simulink model "HSX_multi_fin"  (R2023b)
settings: Solver=VariableStepAuto  StartTime=0.0  StopTime=T_end  RelTol=1e-3
undefined symbols (not defined in the file): Kanti, Ki, Kp, LHSX, Ra, RHSX, T_trigger, Tdead, Ts, Tsamp, Vf
libraries: spsCurrentMeasurementLib x6, spsVoltageMeasurementLib x6, spsSeriesRLCBranchLib x6, spsMosfetLib x4, spsControlledVoltageSourceLib x2, spsDCMachineLib x2, spsSawtoothGeneratorLib x2, spsGroundLib x2, spsIdealSwitchLib x2, spsDCVoltageSourceLib x2, spsDiodeLib x1, sps_lib x1
settings Model: Creator=baik3-ad  LastModifiedBy=baik3-ad

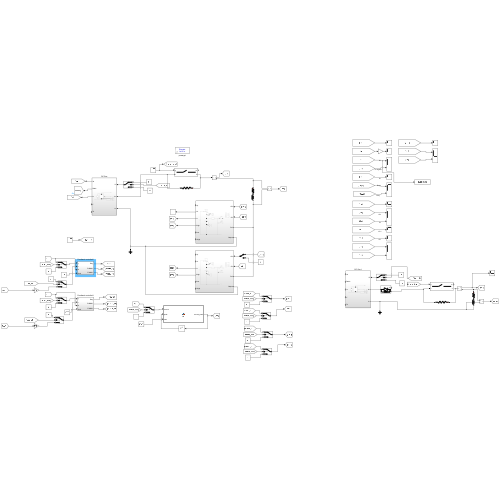
[thumbnail: Simulink's stored preview of the top-level diagram]
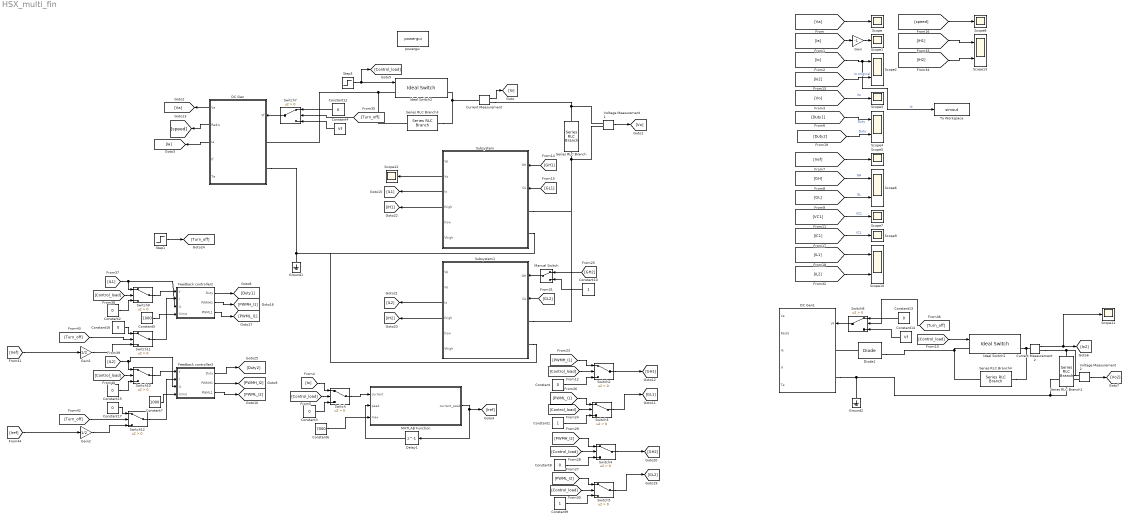
== system HSX_multi_fin ==
  Constant{,2..3,8,12..13,15..17} (9 alike) : Constant  Value=0
  Constant1 : Constant
  Constant10 : Constant
  Constant14 : Constant  Value=Vf
  Constant4 : Constant  Value=Vf
  Constant5 : Constant  Value=1000
  Constant6 : Constant  Value=7000
  Constant7 : Constant  Value=1000
  Constant9 : Constant
  Current Measurement : spsCurrentMeasurementLib/Current Measurement  PhasorSimulation=off  OutputType=Complex  PSBequivalent=0
  Current Measurement2 : spsCurrentMeasurementLib/Current Measurement  PhasorSimulation=off  OutputType=Complex  PSBequivalent=0
  DC Gen : Subsystem
  DC Gen1 : Subsystem
  Delay1 : Delay  DelayLength=1  InitialCondition=0  SampleTime=Tsamp
  Diode1 : spsDiodeLib/Diode  Ron=0.001  Lon=0  Vf=0.8  IC=0  UseSnubber=0  Rs=500  Cs=250e-9  Measurements=on
  Feedback controller2 : Subsystem
  Feedback controller3 : Subsystem
  Gain : Gain  Gain=-1
  Gain1 : Gain  Gain=1/2
  Gain2 : Gain  Gain=1/2
  Ground1 : spsGroundLib/Ground  LConnTagsString=a
  Ground2 : spsGroundLib/Ground  LConnTagsString=a
  Ideal Switch1 : spsIdealSwitchLib/Ideal Switch  Ron=1e-6  Lon=0  IC=0  Rs=1e8  Cs=0  Measurements=on
  Ideal Switch2 : spsIdealSwitchLib/Ideal Switch  Ron=1e-6  Lon=0  IC=0  Rs=1e8  Cs=0  Measurements=on
  MATLAB Function : MATLAB Function  TreatAsAtomicUnit=on
  Manual Switch : ManualSwitch
  Scope{,1,3,5,7..9,11..12} (9 alike) : Scope
  Scope{2,4,6,10,13} (5 alike) : Scope  NumInputPorts=2
  Series RLC Branch : spsSeriesRLCBranchLib/Series RLC Branch  LConnTagsString=__new0  RConnTagsString=__new0  BranchType=RL  Resistance=RHSX*10  Inductance=LHSX*10  SetiL0=off  InitialCurrent=0  Capacitance=1e-6  Setx0=off  InitialVoltage=0  Measurements=None
  Series RLC Branch1 : spsSeriesRLCBranchLib/Series RLC Branch  LConnTagsString=__new0  RConnTagsString=__new0  BranchType=RL  Resistance=RHSX*10  Inductance=LHSX*10  SetiL0=off  InitialCurrent=0  Capacitance=1e-6  Setx0=off  InitialVoltage=0  Measurements=None
  Series RLC Branch3 : spsSeriesRLCBranchLib/Series RLC Branch  LConnTagsString=__new0  RConnTagsString=__new0  BranchType=R  Resistance=1e8  Inductance=0  SetiL0=off  InitialCurrent=0  Capacitance=1e-6  Setx0=off  InitialVoltage=0  Measurements=None
  Series RLC Branch4 : spsSeriesRLCBranchLib/Series RLC Branch  LConnTagsString=__new0  RConnTagsString=__new0  BranchType=R  Resistance=1e8  Inductance=0  SetiL0=off  InitialCurrent=0  Capacitance=1e-6  Setx0=off  InitialVoltage=0  Measurements=None
  Step1 : Step  Time=T_trigger+1.5  SampleTime=0  VectorParams1D=off  ZeroCross=off
  Step3 : Step  Time=T_trigger  SampleTime=0  VectorParams1D=off  ZeroCross=off
  Subsystem : Subsystem
  Subsystem1 : Subsystem
  Switch{,2..5,7..12} (11 alike) : Switch  Criteria=u2 > Threshold  SaturateOnIntegerOverflow=off  InputSameDT=off
  To Workspace : ToWorkspace  VariableName=simout  SaveFormat=Timeseries  SampleTime=-1
  Voltage Measurement1 : spsVoltageMeasurementLib/Voltage Measurement  PhasorSimulation=off  OutputType=Complex  PSBequivalent=0
  Voltage Measurement2 : spsVoltageMeasurementLib/Voltage Measurement  PhasorSimulation=off  OutputType=Complex  PSBequivalent=0
  powergui : sps_lib/powergui  Priority=1  SimulationMode=Discrete  SampleTime=Tsamp  frequency=60  Iterations=50  frequencyindice=0  Pbase=100e6  ErrMax=1e-4  UnitsV=kV  UnitsW=MW  buscounter=0  FunctionMessages=off  echomessages=off  EnableUseOfTLC=off  CurrentSourceSwitches=off  DisableSnubberDevices=off  DisableRonSwitches=off  DisableVfSwitches=off  DisplayEquations=off  AutomaticDiscreteSolvers=off  SolverType=Tustin/Backward Euler (TBE)  Interpol=off  ExternalGateDelay=off  methode=off  Ts=100  x0status=blocks  SPID=on  SwTol=0  HookPort=off  NonlinearTolerance=1e-4  nMaxIteration=100  ContinueOnMaxIteration=off  RestoreLinks=warning  ResistiveCurrentMeasurement=off  Frange=[0:2:500]  Ylog=off  Xlog=on  ShowGrid=off  save=off  variable=ZData  structure=0  ZoomFFT=off  StartTime=0.0  cycles=1  DisplayStyle=1  fundamental=60  FreqAxis=off  MaxFrequency=1000  frequencyindicesteady=1  RmsSteady=1  display=off
  wires:
  Step3/1 -> [Control_load], Ideal Switch2/1
  Current Measurement/1 -> [Io]
  Voltage Measurement1/1 -> [Vo]
  [Va] -> Scope/1
  [Io] -> To Workspace/1, Scope2/1  "Io"
  [Vo] -> Scope3/1  "Vo"
  [Ia] -> Gain/1
  Gain/1 -> Scope1/1
  MATLAB Function/1(current_peak) -> [Iref], Delay1/1
  Delay1/1 -> MATLAB Function/2(peak)
  [Iref] -> Scope5/1
  [GH] -> Scope6/1  "GH"
  [GL] -> Scope6/2  "GL"
  [VC1] -> Scope7/1  "VC1"
  Switch2/1 -> [GH1]
  Switch3/1 -> [GL1]
  [speed] -> Scope8/1
  [IC1] -> Scope9/1  "IC1"
  [IL1] -> Scope10/1
  [Control_load] -> Switch/2
  Switch/1 -> MATLAB Function/1(current)
  [Io] -> Switch/1
  Constant3/1 -> Switch/3
  [Control_load] -> Switch2/2
  [PWMH_I1] -> Switch2/1
  Constant/1 -> Switch2/3
  [PWML_I1] -> Switch3/1
  Constant1/1 -> Switch3/3
  [Control_load] -> Switch3/2
  Current Measurement2/1 -> Scope11/1, [Io2]
  Voltage Measurement2/1 -> [Vo2]
  [Control_load] -> Ideal Switch1/1
  [Io2] -> Scope2/2  "Io original"
  [Duty1] -> Scope4/1  "Duty"
  Constant6/1 -> MATLAB Function/3(max)
  Switch7/1 -> DC Gen/1(Vf)
  Subsystem/3(Io) -> [IL1]
  Subsystem/2(Vo) -> Scope12/1
  DC Gen/3(Ia) -> [Ia]
  DC Gen/1(Va) -> [Va]
  DC Gen/2(Rad/s) -> [speed]
  Switch4/1 -> [GH2]
  [Control_load] -> Switch5/2
  Constant9/1 -> Switch5/3
  [Control_load] -> Switch4/2
  [PWML_I2] -> Switch5/1
  [PWMH_I2] -> Switch4/1
  Constant8/1 -> Switch4/3
  Switch5/1 -> [GL2]
  [GH1] -> Subsystem/1(GH)
  [GL1] -> Subsystem/2(GL)
  [GL2] -> Subsystem1/2(GL)
  Manual Switch/1 -> Subsystem1/1(GH)
  Subsystem1/3(Io) -> [IL2]
  [IL2] -> Scope10/2
  [GH2] -> Manual Switch/1
  Constant10/1 -> Manual Switch/2
  [IH1] -> Scope13/1
  [IH2] -> Scope13/2
  Subsystem/4(Ihigh) -> [IH1]
  Subsystem1/4(Ihigh) -> [IH2]
  Constant4/1 -> Switch7/3
  [Turn_off] -> Switch7/2
  Constant12/1 -> Switch7/1
  Constant13/1 -> Switch8/1
  Constant14/1 -> Switch8/3
  [Turn_off] -> Switch8/2
  Switch8/1 -> DC Gen1/1(Vf)
  [Control_load] -> Switch9/2
  [IL1] -> Feedback controller2/3(IL), Switch9/1
  Constant2/1 -> Switch9/3
  Switch9/1 -> Feedback controller2/1(y)
  [IL2] -> Feedback controller3/3(IL), Switch10/1
  [Control_load] -> Switch10/2
  Constant15/1 -> Switch10/3
  Switch10/1 -> Feedback controller3/1(y)
  Gain1/1 -> Switch11/3
  [Turn_off] -> Switch11/2
  Constant16/1 -> Switch11/1
  Switch11/1 -> Feedback controller2/2(r)
  Constant17/1 -> Switch12/1
  Gain2/1 -> Switch12/3
  Switch12/1 -> Feedback controller3/2(r)
  [Turn_off] -> Switch12/2
  [Iref] -> Gain1/1
  [Iref] -> Gain2/1
  Step1/1 -> [Turn_off]
  Feedback controller2/1(Duty) -> [Duty1]
  Feedback controller2/2(PWMH1) -> [PWMH_I1]
  Feedback controller2/3(PWML1) -> [PWML_I1]
  Feedback controller3/2(PWMH1) -> [PWMH_I2]
  Feedback controller3/3(PWML1) -> [PWML_I2]
  Feedback controller3/1(Duty) -> [Duty2]
  [Duty2] -> Scope4/2  "Duty"
  Constant5/1 -> Feedback controller2/4(Ilimit)
  Constant7/1 -> Feedback controller3/4(Ilimit)
  connections:
  DC Gen/LConn2 -- Subsystem1/LConn2 -- Subsystem/LConn2 -- Ground1/LConn1
  Current Measurement/RConn1 -- Voltage Measurement1/LConn1 -- Series RLC Branch/LConn1
  Current Measurement/LConn1 -- Ideal Switch2/RConn1 -- Series RLC Branch3/LConn1
  Ideal Switch1/LConn1 -- Diode1/RConn1 -- Series RLC Branch4/RConn1
  Ideal Switch1/RConn1 -- Current Measurement2/LConn1 -- Series RLC Branch4/LConn1
  Series RLC Branch1/LConn1 -- Voltage Measurement2/LConn1 -- Current Measurement2/RConn1
  Diode1/LConn1 -- DC Gen1/LConn1
  DC Gen1/LConn2 -- Series RLC Branch1/RConn1 -- Voltage Measurement2/LConn2 -- Ground2/LConn1
  Ideal Switch2/LConn1 -- DC Gen/LConn1 -- Series RLC Branch3/RConn1
  Voltage Measurement1/LConn2 -- Subsystem1/LConn1 -- Subsystem/LConn1 -- Series RLC Branch/RConn1

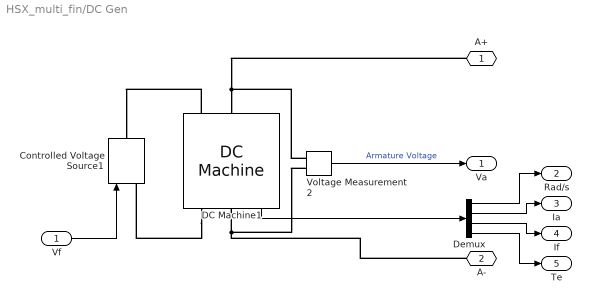
== system HSX_multi_fin/DC Gen ==
  Vf : Inport
  Controlled Voltage Source1 : spsControlledVoltageSourceLib/Controlled Voltage Source  Initialize=on  Source_Type=DC  Amplitude=0  Phase=0  Frequency=0  Measurements=Voltage
  DC Machine1 : spsDCMachineLib/DC Machine  PresetModel=No  MechanicalLoad=Torque TL  FieldType=Wound  ShowDetailedParameters=on  MeasurementBus=off  RLa="[Ra  0.002]"  RLf=[0.0054 0.0125]  Laf=Laf  MachineConstant=Torque constant (N.m/A)  Ke=1.8  Kt=1.8  J=137  Bm=0  Tf=0  w0=w_initial  Ifinit=0  TsPowergui=0  TsBlock=-1
  Demux : Demux
  Voltage Measurement2 : spsVoltageMeasurementLib/Voltage Measurement  PhasorSimulation=off  OutputType=Complex  PSBequivalent=0
  A+ : PMIOPort  Side=Left
  A- : PMIOPort  Port=2  Side=Left
  Va : Outport
  Rad/s : Outport  Port=2
  Ia : Outport  Port=3
  If : Outport  Port=4
  Te : Outport  Port=5
  wires:
  DC Machine1/1 -> Demux/1
  Vf/1 -> Controlled Voltage Source1/1
  Voltage Measurement2/1 -> Va/1  "Armature Voltage"
  Demux/1 -> Rad/s/1
  Demux/4 -> Te/1
  Demux/3 -> If/1
  Demux/2 -> Ia/1
  connections:
  Voltage Measurement2/LConn1 -- A+/RConn1 -- DC Machine1/LConn1
  A-/RConn1 -- Voltage Measurement2/LConn2 -- DC Machine1/RConn1
  DC Machine1/LConn2 -- Controlled Voltage Source1/RConn1
  DC Machine1/RConn2 -- Controlled Voltage Source1/LConn1

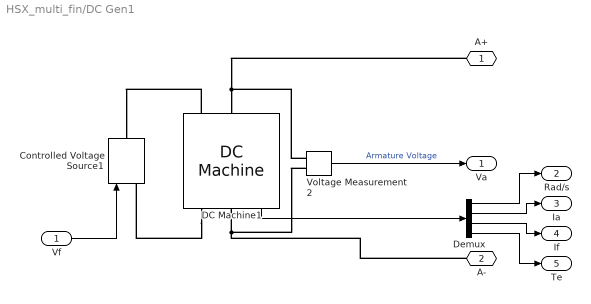
== system HSX_multi_fin/DC Gen1 ==
  Vf : Inport
  Controlled Voltage Source1 : spsControlledVoltageSourceLib/Controlled Voltage Source  Initialize=on  Source_Type=DC  Amplitude=0  Phase=0  Frequency=0  Measurements=Voltage
  DC Machine1 : spsDCMachineLib/DC Machine  PresetModel=No  MechanicalLoad=Torque TL  FieldType=Wound  ShowDetailedParameters=on  MeasurementBus=off  RLa="[Ra  0.002]"  RLf=[0.0054 0.0125]  Laf=Laf  MachineConstant=Torque constant (N.m/A)  Ke=1.8  Kt=1.8  J=137  Bm=0  Tf=0  w0=w_initial  Ifinit=0  TsPowergui=0  TsBlock=-1
  Demux : Demux
  Voltage Measurement2 : spsVoltageMeasurementLib/Voltage Measurement  PhasorSimulation=off  OutputType=Complex  PSBequivalent=0
  A+ : PMIOPort  Side=Left
  A- : PMIOPort  Port=2  Side=Left
  Va : Outport
  Rad/s : Outport  Port=2
  Ia : Outport  Port=3
  If : Outport  Port=4
  Te : Outport  Port=5
  wires:
  DC Machine1/1 -> Demux/1
  Vf/1 -> Controlled Voltage Source1/1
  Voltage Measurement2/1 -> Va/1  "Armature Voltage"
  Demux/1 -> Rad/s/1
  Demux/4 -> Te/1
  Demux/3 -> If/1
  Demux/2 -> Ia/1
  connections:
  Voltage Measurement2/LConn1 -- A+/RConn1 -- DC Machine1/LConn1
  A-/RConn1 -- Voltage Measurement2/LConn2 -- DC Machine1/RConn1
  DC Machine1/LConn2 -- Controlled Voltage Source1/RConn1
  DC Machine1/RConn2 -- Controlled Voltage Source1/LConn1

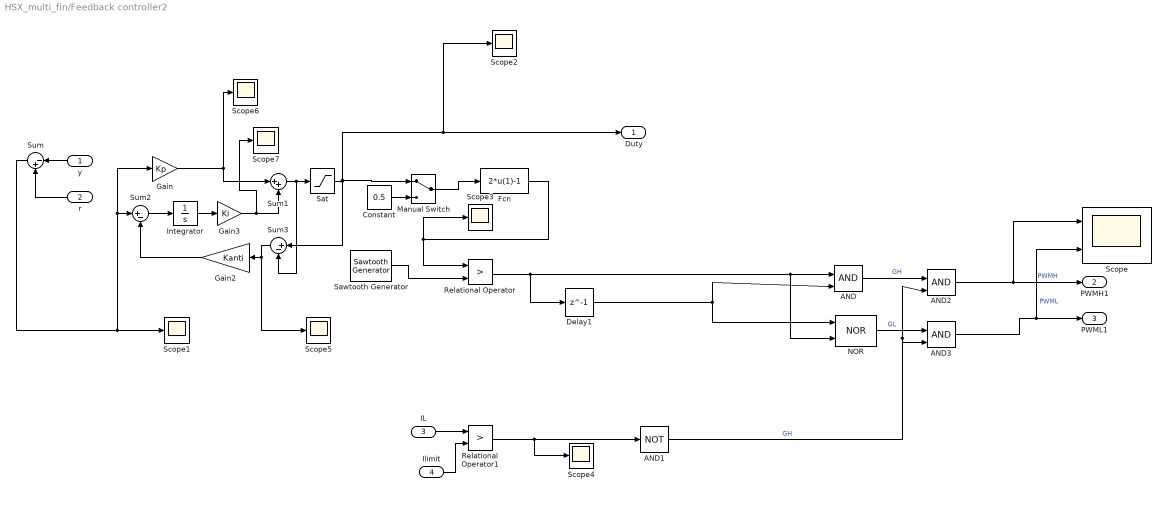
== system HSX_multi_fin/Feedback controller2 ==
  y : Inport
  r : Inport  Port=2
  IL : Inport  Port=3
  Ilimit : Inport  Port=4
  AND : Logic  IconShape=distinctive  AllPortsSameDT=off  OutDataTypeStr=boolean
  AND1 : Logic  Operator=NOT  IconShape=distinctive  AllPortsSameDT=off  OutDataTypeStr=boolean
  AND2 : Logic  IconShape=distinctive  AllPortsSameDT=off  OutDataTypeStr=boolean
  AND3 : Logic  IconShape=distinctive  AllPortsSameDT=off  OutDataTypeStr=boolean
  Constant : Constant  Value=0.5
  Delay1 : Delay  DelayLength=1  InitialCondition=0  SampleTime=Tdead
  Fcn : Fcn  Expr=2*u(1)-1
  Gain : Gain  Gain=Kp
  Gain2 : Gain  Gain=Kanti
  Gain3 : Gain  Gain=Ki
  Integrator : Integrator
  Manual Switch : ManualSwitch
  NOR : Logic  Operator=NOR  IconShape=distinctive  AllPortsSameDT=off
  Relational Operator : RelationalOperator  Operator=>  OutDataTypeStr=boolean  RndMeth=Simplest  InputSameDT=off
  Relational Operator1 : RelationalOperator  Operator=>  OutDataTypeStr=boolean  RndMeth=Simplest  InputSameDT=off
  Sat : Saturate  UpperLimit=1  LowerLimit=0
  Sawtooth Generator : spsSawtoothGeneratorLib/Sawtooth Generator  Freq=1/Ts  Phase=0  Ts=Tsamp
  Scope : Scope  NumInputPorts=2
  Scope{1..7} (7 alike) : Scope
  Sum : Sum  Inputs=|-+  InputSameDT=on  SaturateOnIntegerOverflow=on  OutDataTypeStr=Inherit: Same as first input
  Sum1 : Sum  Inputs=|++
  Sum2 : Sum  Inputs=|+-
  Sum3 : Sum  Inputs=|+-
  Duty : Outport  VectorParamsAs1DForOutWhenUnconnected=off
  PWMH1 : Outport  Port=2  VectorParamsAs1DForOutWhenUnconnected=off
  PWML1 : Outport  Port=3  VectorParamsAs1DForOutWhenUnconnected=off
  wires:
  Sum/1 -> Scope1/1, Gain/1, Sum2/1
  y/1 -> Sum/1
  r/1 -> Sum/2
  Sat/1 -> Sum3/1, Manual Switch/1, Scope2/1, Duty/1
  Sum1/1 -> Sum3/2, Sat/1
  Gain/1 -> Scope6/1, Sum1/1
  Sum2/1 -> Integrator/1
  Sum3/1 -> Scope5/1, Gain2/1
  Gain2/1 -> Sum2/2
  Sawtooth Generator/1 -> Relational Operator/2
  Relational Operator/1 -> Delay1/1, NOR/2, AND/1
  Delay1/1 -> NOR/1, AND/2
  Fcn/1 -> Scope3/1, Relational Operator/1
  Integrator/1 -> Gain3/1
  Gain3/1 -> Scope7/1, Sum1/2
  AND/1 -> AND2/1  "GH"
  AND2/1 -> Scope/1, PWMH1/1  "PWMH"
  AND3/1 -> PWML1/1, Scope/2  "PWML"
  NOR/1 -> AND3/1  "GL"
  Manual Switch/1 -> Fcn/1
  Constant/1 -> Manual Switch/2
  Relational Operator1/1 -> Scope4/1, AND1/1
  Ilimit/1 -> Relational Operator1/2
  IL/1 -> Relational Operator1/1
  AND1/1 -> AND3/2, AND2/2  "GH"

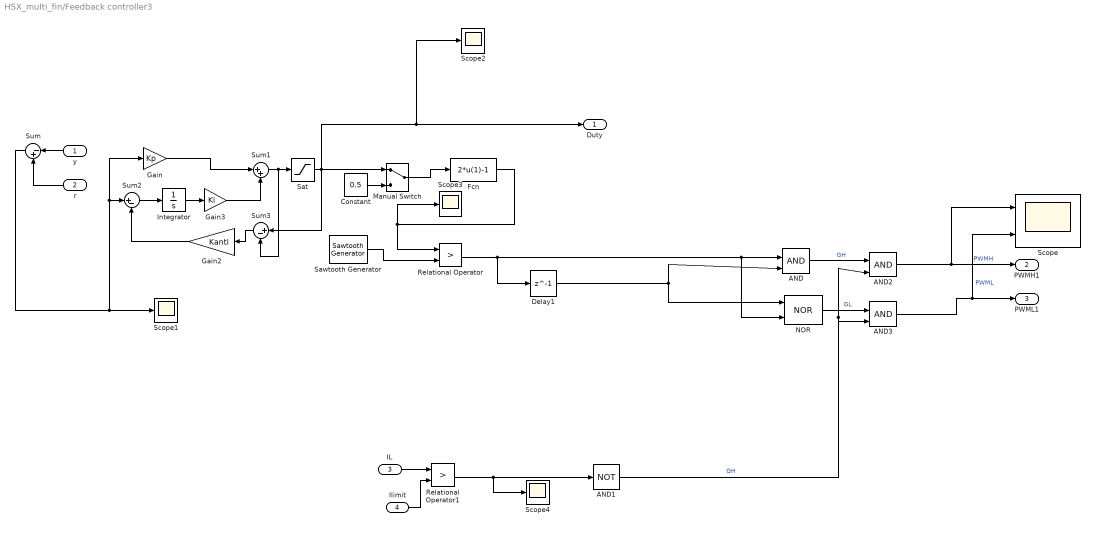
== system HSX_multi_fin/Feedback controller3 ==
  y : Inport
  r : Inport  Port=2
  IL : Inport  Port=3
  Ilimit : Inport  Port=4
  AND : Logic  IconShape=distinctive  AllPortsSameDT=off  OutDataTypeStr=boolean
  AND1 : Logic  Operator=NOT  IconShape=distinctive  AllPortsSameDT=off  OutDataTypeStr=boolean
  AND2 : Logic  IconShape=distinctive  AllPortsSameDT=off  OutDataTypeStr=boolean
  AND3 : Logic  IconShape=distinctive  AllPortsSameDT=off  OutDataTypeStr=boolean
  Constant : Constant  Value=0.5
  Delay1 : Delay  DelayLength=1  InitialCondition=0  SampleTime=Tdead
  Fcn : Fcn  Expr=2*u(1)-1
  Gain : Gain  Gain=Kp
  Gain2 : Gain  Gain=Kanti
  Gain3 : Gain  Gain=Ki
  Integrator : Integrator
  Manual Switch : ManualSwitch
  NOR : Logic  Operator=NOR  IconShape=distinctive  AllPortsSameDT=off
  Relational Operator : RelationalOperator  Operator=>  OutDataTypeStr=boolean  RndMeth=Simplest  InputSameDT=off
  Relational Operator1 : RelationalOperator  Operator=>  OutDataTypeStr=boolean  RndMeth=Simplest  InputSameDT=off
  Sat : Saturate  UpperLimit=1  LowerLimit=0
  Sawtooth Generator : spsSawtoothGeneratorLib/Sawtooth Generator  Freq=1/Ts  Phase=180  Ts=Tsamp
  Scope : Scope  NumInputPorts=2
  Scope{1..4} (4 alike) : Scope
  Sum : Sum  Inputs=|-+  InputSameDT=on  SaturateOnIntegerOverflow=on  OutDataTypeStr=Inherit: Same as first input
  Sum1 : Sum  Inputs=|++
  Sum2 : Sum  Inputs=|+-
  Sum3 : Sum  Inputs=|+-
  Duty : Outport  VectorParamsAs1DForOutWhenUnconnected=off
  PWMH1 : Outport  Port=2  VectorParamsAs1DForOutWhenUnconnected=off
  PWML1 : Outport  Port=3  VectorParamsAs1DForOutWhenUnconnected=off
  wires:
  Sum/1 -> Scope1/1, Gain/1, Sum2/1
  y/1 -> Sum/1
  r/1 -> Sum/2
  Sat/1 -> Sum3/1, Manual Switch/1, Scope2/1, Duty/1
  Sum1/1 -> Sum3/2, Sat/1
  Gain/1 -> Sum1/1
  Sum2/1 -> Integrator/1
  Sum3/1 -> Gain2/1
  Gain2/1 -> Sum2/2
  Sawtooth Generator/1 -> Relational Operator/2
  Relational Operator/1 -> Delay1/1, NOR/2, AND/1
  Delay1/1 -> NOR/1, AND/2
  Fcn/1 -> Scope3/1, Relational Operator/1
  Integrator/1 -> Gain3/1
  Gain3/1 -> Sum1/2
  AND/1 -> AND2/1  "GH"
  AND2/1 -> Scope/1, PWMH1/1  "PWMH"
  AND3/1 -> PWML1/1, Scope/2  "PWML"
  NOR/1 -> AND3/1  "GL"
  Manual Switch/1 -> Fcn/1
  Constant/1 -> Manual Switch/2
  IL/1 -> Relational Operator1/1
  Relational Operator1/1 -> Scope4/1, AND1/1
  Ilimit/1 -> Relational Operator1/2
  AND1/1 -> AND3/2, AND2/2  "GH"

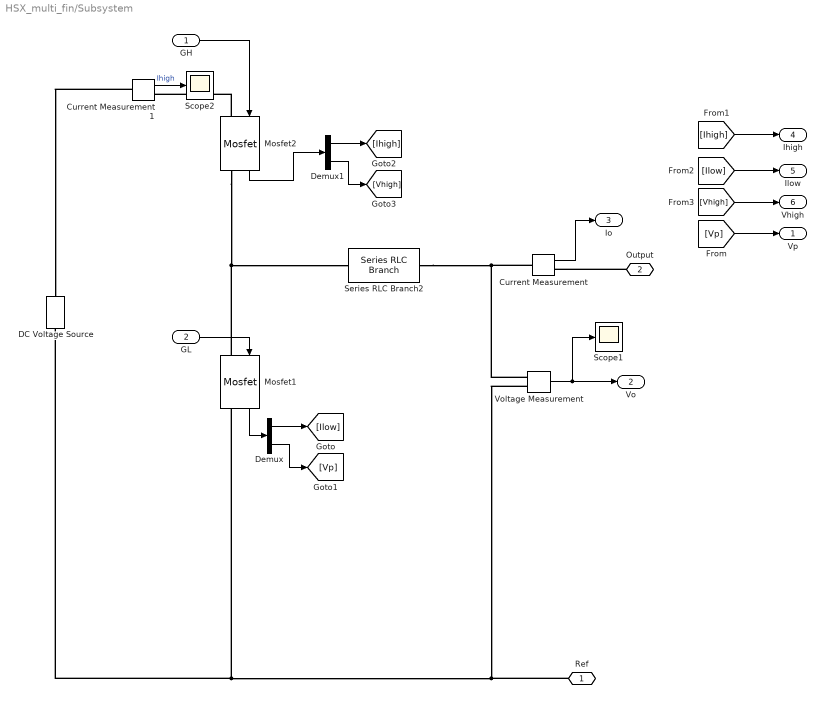
== system HSX_multi_fin/Subsystem ==
  GH : Inport
  GL : Inport  Port=2
  Current Measurement : spsCurrentMeasurementLib/Current Measurement  PhasorSimulation=off  OutputType=Complex  PSBequivalent=0
  Current Measurement1 : spsCurrentMeasurementLib/Current Measurement  PhasorSimulation=off  OutputType=Complex  PSBequivalent=0
  DC Voltage Source : spsDCVoltageSourceLib/DC Voltage Source  Amplitude=50  Measurements=None
  Demux : Demux  Outputs=2
  Demux1 : Demux  Outputs=2
  Mosfet1 : spsMosfetLib/Mosfet  Ron=0.0001  Lon=0  Rd=0.0001  Vfd=0.01  IC=0  Rs=1e5  Cs=inf  Measurements=on
  Mosfet2 : spsMosfetLib/Mosfet  Ron=0.0001  Lon=0  Rd=0.0001  Vfd=0.01  IC=0  Rs=1e5  Cs=inf  Measurements=on
  Scope1 : Scope
  Scope2 : Scope
  Series RLC Branch2 : spsSeriesRLCBranchLib/Series RLC Branch  LConnTagsString=__new0  RConnTagsString=__new0  BranchType=L  Resistance=0.09  Inductance=1e-3  SetiL0=on  InitialCurrent=0  Capacitance=1e-1  Setx0=off  InitialVoltage=0  Measurements=None
  Voltage Measurement : spsVoltageMeasurementLib/Voltage Measurement  PhasorSimulation=off  OutputType=Complex  PSBequivalent=0
  Ref : PMIOPort  Side=Left
  Output : PMIOPort  Port=2  Side=Left
  Vp : Outport
  Vo : Outport  Port=2
  Io : Outport  Port=3
  Ihigh : Outport  Port=4
  Ilow : Outport  Port=5
  Vhigh : Outport  Port=6
  wires:
  Voltage Measurement/1 -> Vo/1, Scope1/1
  GL/1 -> Mosfet1/1
  Current Measurement/1 -> Io/1
  Mosfet1/1 -> Demux/1
  Demux/1 -> [Ilow]
  Demux/2 -> [Vp]
  [Vp] -> Vp/1
  GH/1 -> Mosfet2/1
  Demux1/2 -> [Vhigh]
  Mosfet2/1 -> Demux1/1
  Demux1/1 -> [Ihigh]
  [Ihigh] -> Ihigh/1
  [Ilow] -> Ilow/1
  [Vhigh] -> Vhigh/1
  Current Measurement1/1 -> Scope2/1  "Ihigh"
  connections:
  Series RLC Branch2/RConn1 -- Current Measurement/LConn1 -- Voltage Measurement/LConn1
  Mosfet1/LConn1 -- Mosfet2/RConn1 -- Series RLC Branch2/LConn1
  Voltage Measurement/LConn2 -- DC Voltage Source/LConn1 -- Mosfet1/RConn1 -- Ref/RConn1
  Output/RConn1 -- Current Measurement/RConn1
  Current Measurement1/LConn1 -- DC Voltage Source/RConn1
  Mosfet2/LConn1 -- Current Measurement1/RConn1

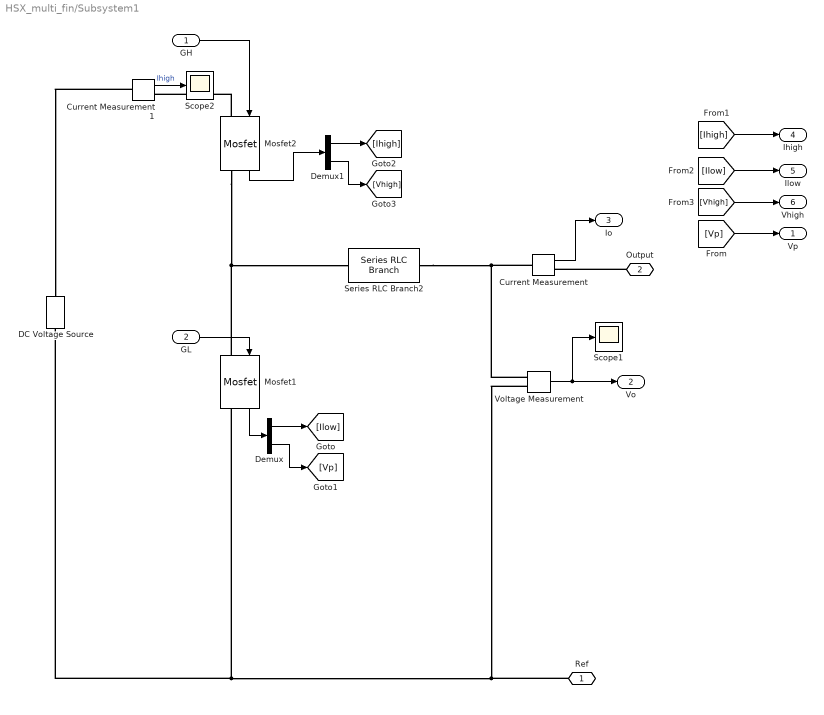
== system HSX_multi_fin/Subsystem1 ==
  GH : Inport
  GL : Inport  Port=2
  Current Measurement : spsCurrentMeasurementLib/Current Measurement  PhasorSimulation=off  OutputType=Complex  PSBequivalent=0
  Current Measurement1 : spsCurrentMeasurementLib/Current Measurement  PhasorSimulation=off  OutputType=Complex  PSBequivalent=0
  DC Voltage Source : spsDCVoltageSourceLib/DC Voltage Source  Amplitude=50  Measurements=None
  Demux : Demux  Outputs=2
  Demux1 : Demux  Outputs=2
  Mosfet1 : spsMosfetLib/Mosfet  Ron=0.0001  Lon=0  Rd=0.0001  Vfd=0.01  IC=0  Rs=1e5  Cs=inf  Measurements=on
  Mosfet2 : spsMosfetLib/Mosfet  Ron=0.0001  Lon=0  Rd=0.0001  Vfd=0.01  IC=0  Rs=1e5  Cs=inf  Measurements=on
  Scope1 : Scope
  Scope2 : Scope
  Series RLC Branch2 : spsSeriesRLCBranchLib/Series RLC Branch  LConnTagsString=__new0  RConnTagsString=__new0  BranchType=L  Resistance=0.09  Inductance=1e-3  SetiL0=on  InitialCurrent=0  Capacitance=1e-1  Setx0=off  InitialVoltage=0  Measurements=None
  Voltage Measurement : spsVoltageMeasurementLib/Voltage Measurement  PhasorSimulation=off  OutputType=Complex  PSBequivalent=0
  Ref : PMIOPort  Side=Left
  Output : PMIOPort  Port=2  Side=Left
  Vp : Outport
  Vo : Outport  Port=2
  Io : Outport  Port=3
  Ihigh : Outport  Port=4
  Ilow : Outport  Port=5
  Vhigh : Outport  Port=6
  wires:
  Voltage Measurement/1 -> Vo/1, Scope1/1
  GL/1 -> Mosfet1/1
  Current Measurement/1 -> Io/1
  Mosfet1/1 -> Demux/1
  Demux/1 -> [Ilow]
  Demux/2 -> [Vp]
  [Vp] -> Vp/1
  GH/1 -> Mosfet2/1
  Demux1/2 -> [Vhigh]
  Mosfet2/1 -> Demux1/1
  Demux1/1 -> [Ihigh]
  [Ihigh] -> Ihigh/1
  [Ilow] -> Ilow/1
  [Vhigh] -> Vhigh/1
  Current Measurement1/1 -> Scope2/1  "Ihigh"
  connections:
  Series RLC Branch2/RConn1 -- Current Measurement/LConn1 -- Voltage Measurement/LConn1
  Mosfet2/RConn1 -- Mosfet1/LConn1 -- Series RLC Branch2/LConn1
  Voltage Measurement/LConn2 -- DC Voltage Source/LConn1 -- Mosfet1/RConn1 -- Ref/RConn1
  Output/RConn1 -- Current Measurement/RConn1
  Current Measurement1/LConn1 -- DC Voltage Source/RConn1
  Mosfet2/LConn1 -- Current Measurement1/RConn1

== matlab function HSX_multi_fin/MATLAB Function ==
  data: current input; current_peak output; peak input; max input
function current_peak = fcn(current, peak,max)
    if current>peak
        current_peak = current;
    else
        current_peak = peak;
    end

    if (max ~= 0)&&(peak>=max)
        current_peak = max;
     
    end
